simulink model "tilted_hysteresis"  (R2015a)
settings: Solver=ode45  StartTime=0.0  StopTime=3  RelTol=1e-3
settings Model: Creator=RAK  LastModifiedBy=RAK

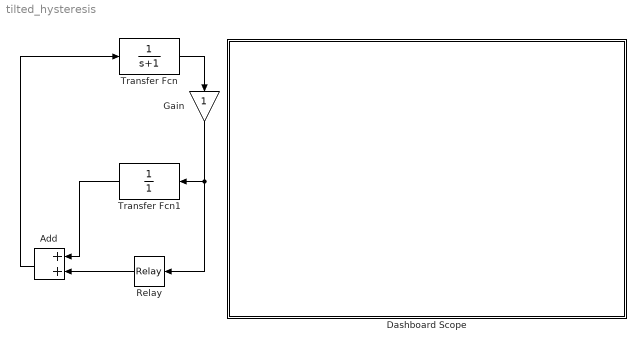
== system tilted_hysteresis ==
  Add : Sum
  Dashboard Scope : Subsystem  DialogController=hmiCreateDDGDialog  IsWebBlock=on  mask(MathWorksWebBlock){webBlockId=85c96e75-d4f5-4be1-8d8d-f0b9f3f843f4, webBlockType=sdiscope, ShowInitialText=on, HMISrcModelName=tilted_hysteresis}
      mask prompts: webBlockId "WebBlock Id"; webBlockType "WebBlock Type"; HMISrcModelName "Source Model"
      mask Help: helpview([docroot '/mapfiles/simulink.map'], 'hmi_scope')
      mask Display:
      | if strcmp(get_param(bdroot(gcb),'BlockDiagramType'), 'library')
      |     image([(matlabroot) '/toolbox/simulink/hmi/icons/DashboardScope.png']);
      | end
  Gain : Gain
  Relay : Relay  OnSwitchValue=0.6262  OffSwitchValue=0.4976  OnOutputValue=-.2829  OffOutputValue=.98640
  Transfer Fcn : TransferFcn  Denominator=[1 1]
  Transfer Fcn1 : TransferFcn  Numerator=1  Denominator=[1]
  wires:
  Relay/1 -> Add/2
  Transfer Fcn1/1 -> Add/1
  Add/1 -> Transfer Fcn/1
  Transfer Fcn/1 -> Gain/1
  Gain/1 -> Relay/1, Transfer Fcn1/1

== system tilted_hysteresis/Dashboard Scope ==
